simulink model "s32k3_summerschool_base"  (R2026a)
settings: Solver=FixedStepAuto  FixedStep=0.1  EnableMultiTasking=on
PreLoadFcn:
  | % NXP_MBDT_S32K3 callback: DO NOT REMOVE
  | mbd_s32k3.common.nxp.model_callbacks.preLoadFcn();
PostLoadFcn:
  | % NXP_MBDT_S32K3 callback: DO NOT REMOVE
  | mbd_s32k3.common.nxp.model_callbacks.postLoadFcn();
InitFcn:
  | % NXP_MBDT_S32K3 callback: DO NOT REMOVE
  | mbd_s32k3.common.nxp.model_callbacks.initFcn();
libraries: mbd_s32k3_io_library x12, mbd_s32k3_isr_library x2, mbd_s32k3_utility_library x1
Description:
  | Dio S32CT
  | 
  | 
  |             <script src="../../../doc/src/utils.js">
  | 
  |             <script src="../../../doc/src/details_summary_utils.js">
  | 
  |             <script src="../../../doc/src/matlab_command_link.js">
  | 
  |             <link rel="stylesheet" type="text/css" href="../../../doc/style.css">
  | 
  | 
  | 
  | 
  |         Dio S32CT
  |         <a class="matlab-command" href="matlab:mbd_s32k3.nxp.openexample('s32k3_summerschool_base')"><button class="matlab-command" style=" --data-title: ' Run MATLAB command: mbd_s32k3.nxp.openexample (\'s32k3_summerschool_base\')'">Open Example
  |         The s32k3_summerschool_base.mdl example shows how to use DIO ReadChannel, WriteChannel and FlipChannel functionalities.
  | 
  |             The application consists of 3 Dio blocks: FlipChannel, ReadChannel and WriteChannel. FlipChannel block is used to toggle DioLed0. The state of DioLed0 is stored inside the red_led_level variable. ReadChannel block is used to toggle the switch DioButton0 and is correlated with WriteChannel block which is used to toggle DioLed2.
  | 
  |             The versionInfo variable stores the version information of this module, including module id, vendor id and vendor specific version numbers.
  | 
  |             Note: the default settings of initialization for the peripherals used in this example represent just a default S32 Configuration Tools available configuration.Users can change the configuration structure's setting in application to fit the special requirement.If you would like to change the configuration tool, please follow the steps described in the Customization Options section.
  | 
  |         Toolchain Supported
  | 
  | 
  |                 S32 Design Studio 3.6.4
  | 
  | 
  |         Required Hardware
  | 
  | 
  |                 Personal Computer
  | 
  |                 S32K311EVB-Q100 / S32K312EVB-Q172 / S32K312MINI-EVB / S32K3X4EVB-Q172 / S32K3X4EVB-T172 / S32K3X4EVB-Q257 / S32K388EVB-Q289 / S32K389EVB-Q437 / XS32K396-BGA-DC (compatible with S32K374, S32K376, S32K394 and S32K396 MCUs) board
  | 
  |                 12V Power Supply
  | 
  |                 Micro USB cable
  | 
  | 
  |         Prepare the Demo
  | 
  | 
  |                 Open the model and select the processor package. This model is configured for the S32K344-Q257 hardware part. If you would like to change the processor package, please follow the steps described in the Customization Options section.
  | 
  |                 Connect an USB cable between the host PC and the OpenSDA USB port on the EVB. In case the OpenSDA port is not available, an external probe (P&E Micro Multilink) can be used.
  | 
  |                 Build and Download the program on the target MCU.
  | 
  | 
  |         Running the Demo
  | 
  | 
  |                 After the application is deployed on target, the DioLed0 should blink every 0.1 second. If DioButton0 is pressed, the DioLed2 should turn on.
  | 
  |                 The following table provides a mapping between the configured DIO channels and the available hardware pins: <table class="tg">S32K3X4EVB-Q257S32K388EVB-Q289S32K311EVB-Q100S32K312EVB-Q172S32K3X4EVB-Q172S32K3X4EVB-T172XS32K396-BGA-DCXS32K396-BGA-DC1MR-CANHUBK344S32K344EVB-WBDioLed0RGBLED0_REDRGBLED0_REDRGBLED0_REDRGBLED0_REDRGBLED0_REDRGBLED0_REDD33_BLUED33_BLUERGBLED0_GREEND28_GREENDioLed1RGBLED0_GREENRGBLED0_GREENRGBLED0_GREENRGBLED0_GREENRGBLED0_GREENRGBLED0_GREEND34_BLUED34_BLUERGBLED0_BLUED29_GREENDioLed2RGBLED0_BLUERGBLED0_BLUERGBLED0_BLUERGBLED0_BLUERGBLED0_BLUERGBLED0_BLUED35_BLUED35_BLUELED_CAN0D30_GREENDioLed3RGBLED1_REDRGBLED1_REDLED_CAN1D31_GREENDioLed4RGBLED1_GREENRGBLED1_GREENDioLed5RGBLED1_BLUERGBLED1_BLUEDioButton0USER_SW0USER_SW0USER_SW0USER_SW0USER_SW0USER_SW0USER_SW7USER_SW7USER_SW1USER_SW2DioButton1USER_SW1USER_SW1USER_SW1USER_SW1USER_SW1USER_SW1USER_SW8USER_SW8USER_SW2USER_SW3DioButton2TOUCH_GPIO_AUSER_SW9USER_SW9DioButton3TOUCH_GPIO_B
  | 
  |                 Note: For configurations using the S32K312MINI-EVB - The LED control via DIO channels uses inverted logic (1 = OFF, 0 = ON).
  | 
  | 
  |         Customization Options
  | 
  | 
  |                 For changing the processor, the configuration tool, and for creating custom configuration projects, please visit the User Manual: <a class="pdf-link" href="../../../doc/docs/manual/SW32K3_MBDT_1.8.0_D2512_UserManual.pdf">SW32K3_MBDT_1.8.0_D2512_UserManual.pdf
  | 
  |                 For S32K3 Design Tools and Files, please visit <a href="https://www.nxp.com/products/processors-and-microcontrollers/arm-microcontrollers/s32k-automotive-mcus/s32k3-microcontrollers-for-general-purpose:S32K3">S32K3 Microcontrollers
  | 
  |                 Fully customizable for any input and output pins using S32 Configuration Tools.
settings Model: DataDictionary=s32k3_summerschool_base.sldd  Creator=nxa06644  LastModifiedBy=nxf64875
settings DebuggingCC: InheritedTsInSrcMsg=none
settings HardwareCC: ProdLargestAtomicInteger=Long  ProdLargestAtomicFloat=Double  ProdHWDeviceType=ARM Compatible->ARM Cortex
settings RTWCC: SystemTargetFile=ert.tlc  HardwareBoard=NXP S32K3xx  TLCOptions=-aInlineSetEventsForThisBaseRateFcn=TLC_FALSE -aSuppressMultiTaskScheduler=TLC_FALSE -aRateBasedStepFcn=1  GenerateReport=on  Toolchain=S32DS GCC  BuildConfiguration=Specify  IncludeHyperlinkInReport=on  LaunchReport=on  GenerateTraceInfo=on  GenerateTraceReport=on  GenerateTraceReportSl=on  GenerateTraceReportSf=on  GenerateTraceReportEml=on  Description=Embedded Coder
settings ERTTargetCC: ERTSrcFileBannerTemplate=mbd_s32k3_ert_code_template.cgt  ERTHdrFileBannerTemplate=mbd_s32k3_ert_code_template.cgt  ERTDataSrcFileTemplate=mbd_s32k3_ert_code_template.cgt  ERTDataHdrFileTemplate=mbd_s32k3_ert_code_template.cgt  DynamicArrayContainerType=coder::array

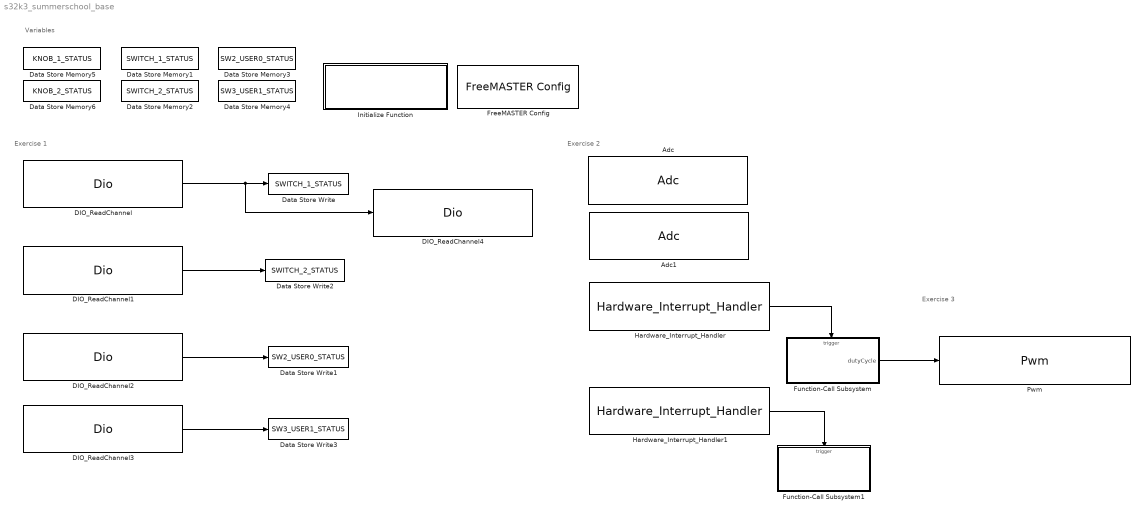
== system s32k3_summerschool_base ==
  note: Exercise 3
  note: Exercise 2
  note: Exercise 1
  note: Variables
  Adc : mbd_s32k3_io_library/Adc  api_func=Adc_StartGroupConversion  hw_unit=AdcHwUnit_0  group=AdcGroup_0  channel=AdcChannel_KNOB_1  threshold_control=No ADC threshold control configured  power_state=ADC_FULL_POWER  ctu_unit=No CTU Unit configured  ctu_trigger=AdcHwTrigger_0  ctu_fifo_idx=No CTU FIFO available  text=<binary blob, 12330 chars, not shown>
      settings: SourceProductName=IO Blocks
  Adc1 : mbd_s32k3_io_library/Adc  api_func=Adc_StartGroupConversion  hw_unit=AdcHwUnit_0  group=AdcGroup_1  channel=AdcChannel_KNOB_1  threshold_control=No ADC threshold control configured  power_state=ADC_FULL_POWER  ctu_unit=No CTU Unit configured  ctu_trigger=AdcHwTrigger_0  ctu_fifo_idx=No CTU FIFO available  text=<binary blob, 12330 chars, not shown>
      settings: SourceProductName=IO Blocks
  DIO_ReadChannel : mbd_s32k3_io_library/Dio  Priority=0  api_func=Dio_ReadChannel  channel=SWITCH_1  channel_group=No channel groups configured  port=PTA_H  gpioSim=off  text=<binary blob, 2169 chars, not shown>
      settings: SourceProductName=IO Blocks
  DIO_ReadChannel1 : mbd_s32k3_io_library/Dio  Priority=0  api_func=Dio_ReadChannel  channel=SWITCH_2  channel_group=No channel groups configured  port=PTA_H  gpioSim=off  text=<binary blob, 2169 chars, not shown>
      settings: SourceProductName=IO Blocks
  DIO_ReadChannel2 : mbd_s32k3_io_library/Dio  Priority=0  api_func=Dio_ReadChannel  channel=SW2_USER0  channel_group=No channel groups configured  port=PTA_H  gpioSim=off  text=<binary blob, 2169 chars, not shown>
      settings: SourceProductName=IO Blocks
  DIO_ReadChannel3 : mbd_s32k3_io_library/Dio  Priority=0  api_func=Dio_ReadChannel  channel=SW3_USER1  channel_group=No channel groups configured  port=PTA_H  gpioSim=off  text=<binary blob, 2169 chars, not shown>
      settings: SourceProductName=IO Blocks
  DIO_ReadChannel4 : mbd_s32k3_io_library/Dio  Priority=0  api_func=Dio_WriteChannel  channel=FAN  channel_group=No channel groups configured  port=PTA_H  gpioSim=off  text=<binary blob, 2169 chars, not shown>
      settings: SourceProductName=IO Blocks
  Data Store Memory1 : DataStoreMemory  DataStoreName=SWITCH_1_STATUS  ReadBeforeWriteMsg=warning  WriteAfterWriteMsg=warning  WriteAfterReadMsg=warning  ShowAdditionalParam=off  OutDataTypeStr=uint8
  Data Store Memory2 : DataStoreMemory  DataStoreName=SWITCH_2_STATUS  ReadBeforeWriteMsg=warning  WriteAfterWriteMsg=warning  WriteAfterReadMsg=warning  ShowAdditionalParam=off  OutDataTypeStr=uint8
  Data Store Memory3 : DataStoreMemory  DataStoreName=SW2_USER0_STATUS  ReadBeforeWriteMsg=warning  WriteAfterWriteMsg=warning  WriteAfterReadMsg=warning  ShowAdditionalParam=off  OutDataTypeStr=uint8
  Data Store Memory4 : DataStoreMemory  DataStoreName=SW3_USER1_STATUS  ReadBeforeWriteMsg=warning  WriteAfterWriteMsg=warning  WriteAfterReadMsg=warning  ShowAdditionalParam=off  OutDataTypeStr=uint8
  Data Store Memory5 : DataStoreMemory  DataStoreName=KNOB_1_STATUS  ReadBeforeWriteMsg=warning  WriteAfterWriteMsg=warning  WriteAfterReadMsg=warning  ShowAdditionalParam=off  OutDataTypeStr=uint16
  Data Store Memory6 : DataStoreMemory  DataStoreName=KNOB_2_STATUS  ReadBeforeWriteMsg=warning  WriteAfterWriteMsg=warning  WriteAfterReadMsg=warning  ShowAdditionalParam=off  OutDataTypeStr=uint16
  Data Store Write : DataStoreWrite  DataStoreName=SWITCH_1_STATUS  IndexOptions=Index vector (dialog)  Indices=1  OutputSizes=1
  Data Store Write1 : DataStoreWrite  DataStoreName=SW2_USER0_STATUS  IndexOptions=Index vector (dialog)  Indices=1  OutputSizes=1
  Data Store Write2 : DataStoreWrite  DataStoreName=SWITCH_2_STATUS  IndexOptions=Index vector (dialog)  Indices=1  OutputSizes=1
  Data Store Write3 : DataStoreWrite  DataStoreName=SW3_USER1_STATUS  IndexOptions=Index vector (dialog)  Indices=1  OutputSizes=1
  FreeMASTER Config : mbd_s32k3_utility_library/FreeMASTER blocks/FreeMASTER Config  connection_type=Serial  instance=LPUART_6  baudrate=115200  isr_prio=5  cantxid=0x7aa  cantxidext=on  cantxobj=5  canrxid=0x7aa  canrxidext=on  canrxobj=5  mode=Short Interrupt  scope_use=1  scope_max_vars=8  automatic_buff_size=on  buff_size=255  default_rfifo_size=on  rfifo_size=32
      settings: SourceProductName=Utility Blocks
  Function-Call Subsystem : Subsystem  TreatAsAtomicUnit=on
  Function-Call Subsystem1 : Subsystem  TreatAsAtomicUnit=on
  Hardware_Interrupt_Handler : mbd_s32k3_isr_library/Hardware_Interrupt_Handler  blockCbk=0  irqGroup=Adc  irqHandlers=Adc_Adc0Group0Notification  irqSim=off  text=<binary blob, 12330 chars, not shown>
      settings: SourceProductName=ISR Blocks
  Hardware_Interrupt_Handler1 : mbd_s32k3_isr_library/Hardware_Interrupt_Handler  blockCbk=0  irqGroup=Adc  irqHandlers=Adc_Adc0Group1Notification  irqSim=off  text=<binary blob, 12330 chars, not shown>
      settings: SourceProductName=ISR Blocks
  Initialize Function : Subsystem  TreatAsAtomicUnit=on
  Pwm : mbd_s32k3_io_library/Pwm  api_func=Pwm_SetDutyCycle  channel=PwmChannel_0  notification=PWM_RISING_EDGE  moduleId=PWM_EMIOS_INSTANCE_0  prescalerType=PWM_PRIMARY_PRESCALER  fault=PWM_FLEXPWM_0_FAULT_INPUT_0  text=<binary blob, 3846 chars, not shown>
      settings: SourceProductName=IO Blocks
  wires:
  DIO_ReadChannel/1 -> DIO_ReadChannel4/1, Data Store Write/1
  DIO_ReadChannel1/1 -> Data Store Write2/1
  DIO_ReadChannel2/1 -> Data Store Write1/1
  DIO_ReadChannel3/1 -> Data Store Write3/1
  Hardware_Interrupt_Handler/1 -> Function-Call Subsystem/Trigger
  Hardware_Interrupt_Handler1/1 -> Function-Call Subsystem1/Trigger
  Function-Call Subsystem/1(dutyCycle) -> Pwm/1

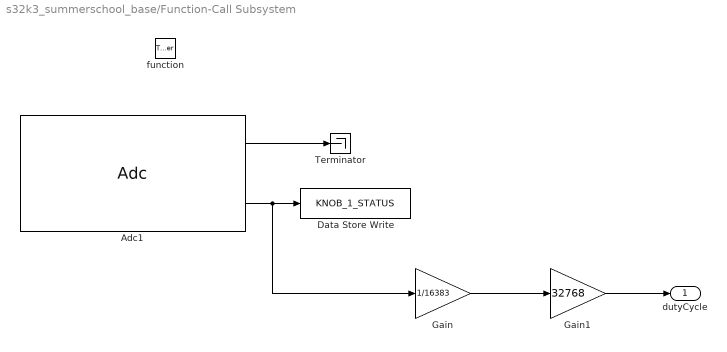
== system s32k3_summerschool_base/Function-Call Subsystem ==
  function : TriggerPort  TriggerType=function-call  VariantControl=(inherit)
  Adc1 : mbd_s32k3_io_library/Adc  api_func=Adc_ReadGroup  hw_unit=AdcHwUnit_0  group=AdcGroup_0  channel=AdcChannel_KNOB_1  threshold_control=No ADC threshold control configured  power_state=ADC_FULL_POWER  ctu_unit=No CTU Unit configured  ctu_trigger=AdcHwTrigger_0  ctu_fifo_idx=No CTU FIFO available  text=<binary blob, 12330 chars, not shown>
      settings: SourceProductName=IO Blocks
  Data Store Write : DataStoreWrite  DataStoreName=KNOB_1_STATUS  IndexOptions=Index vector (dialog)  Indices=1  OutputSizes=1
  Gain : Gain  Gain=1/16383  OutDataTypeStr=single
  Gain1 : Gain  Gain=32768  OutDataTypeStr=uint16
  Terminator : Terminator
  dutyCycle : Outport
  wires:
  Adc1/2 -> Gain/1, Data Store Write/1
  Adc1/1 -> Terminator/1
  Gain/1 -> Gain1/1
  Gain1/1 -> dutyCycle/1

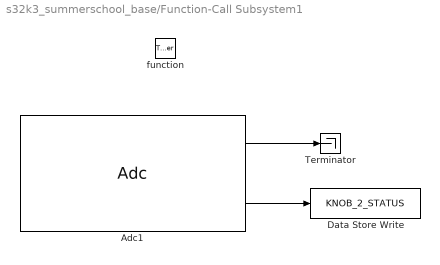
== system s32k3_summerschool_base/Function-Call Subsystem1 ==
  function : TriggerPort  TriggerType=function-call  VariantControl=(inherit)
  Adc1 : mbd_s32k3_io_library/Adc  api_func=Adc_ReadGroup  hw_unit=AdcHwUnit_0  group=AdcGroup_1  channel=AdcChannel_KNOB_1  threshold_control=No ADC threshold control configured  power_state=ADC_FULL_POWER  ctu_unit=No CTU Unit configured  ctu_trigger=AdcHwTrigger_0  ctu_fifo_idx=No CTU FIFO available  text=<binary blob, 12330 chars, not shown>
      settings: SourceProductName=IO Blocks
  Data Store Write : DataStoreWrite  DataStoreName=KNOB_2_STATUS  IndexOptions=Index vector (dialog)  Indices=1  OutputSizes=1
  Terminator : Terminator
  wires:
  Adc1/2 -> Data Store Write/1
  Adc1/1 -> Terminator/1

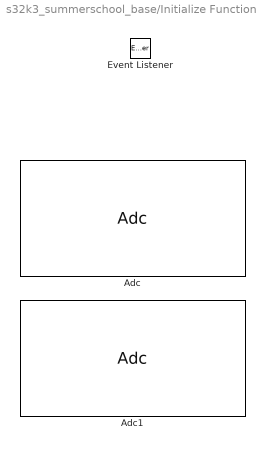
== system s32k3_summerschool_base/Initialize Function ==
  Adc : mbd_s32k3_io_library/Adc  api_func=Adc_EnableGroupNotification  hw_unit=AdcHwUnit_0  group=AdcGroup_0  channel=AdcChannel_KNOB_1  threshold_control=No ADC threshold control configured  power_state=ADC_FULL_POWER  ctu_unit=No CTU Unit configured  ctu_trigger=AdcHwTrigger_0  ctu_fifo_idx=No CTU FIFO available  text=<binary blob, 12330 chars, not shown>
      settings: SourceProductName=IO Blocks
  Adc1 : mbd_s32k3_io_library/Adc  api_func=Adc_EnableGroupNotification  hw_unit=AdcHwUnit_0  group=AdcGroup_1  channel=AdcChannel_KNOB_1  threshold_control=No ADC threshold control configured  power_state=ADC_FULL_POWER  ctu_unit=No CTU Unit configured  ctu_trigger=AdcHwTrigger_0  ctu_fifo_idx=No CTU FIFO available  text=<binary blob, 12330 chars, not shown>
      settings: SourceProductName=IO Blocks
  Event Listener : EventListener  DisableCoverage=on  EventName=reset
